simulink library "eventsBswLib"  (R2023b)
settings: Solver=VariableStepAuto  StartTime=0.0  StopTime=10.0  RelTol=1e-3
libraries: simulink x3, events_bswapi x2
settings Model: Creator=Professional  LastModifiedBy=zon07
settings SFSimCC: SimAnalyzeCustomCode=on  SimTargetLang=C++
settings RTWCC: RTWUseSimCustomCode=on

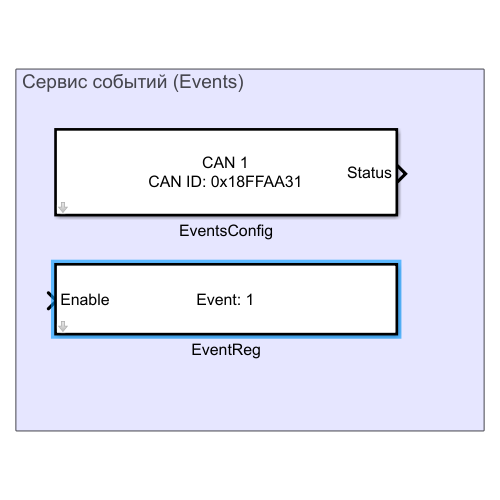
[thumbnail: Simulink's stored preview of the top-level diagram]
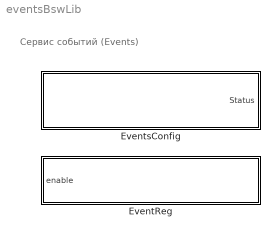
== system eventsBswLib ==
  note: Сервис событий (Events)
  EventReg : Subsystem  TreatAsAtomicUnit=on  mask(Event Registration){eventNum=1}
      mask prompts: eventNum "Номер ивента:"
      mask help:
      | Зарегистрировать ивент.
      | Активация события происходит по изменению enable из false -> true;
      | Сообщение с событием отправиться один раз.
      | Для повторной регистрации события необходимо заново перевести enable из false -> true.
      mask init:
      | blockName = "Event: " + num2str(eventNum);
      mask DialogControl Container2 Prompt: Параметры
      mask Display:
      | disp(blockName);
      | port_label('input', 1, 'Enable');
  EventsConfig : Subsystem  TreatAsAtomicUnit=on  mask(Config Events CanId){can=CAN1, canId=0x18FFAA31}
      mask prompts: canId "Events msg CanId:"
      mask help: Установить CAN ID для отправки ивентов (событий).
      mask init:
      | blockName = "CAN " + can + "\n" + "CAN ID: 0x" + dec2hex(canId);
      mask TypeOptions can: CAN1 | CAN2
      mask DialogControl ParameterGroupVar Prompt: Параметры
      mask Display:
      | disp(blockName);
      | port_label('output', 1, 'Status');

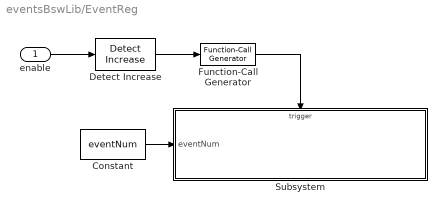
== system eventsBswLib/EventReg ==
  enable : Inport  OutDataTypeStr=boolean
  Constant : Constant  Value=eventNum  OutDataTypeStr=uint16
  Detect Increase : simulink/Logic and Bit Operations/Detect Increase  vinit=0.0  OutDataTypeStr=boolean
  Function-Call Generator : simulink/Ports & Subsystems/Function-Call Generator  sample_time=1  numberOfIterations=1  DisallowWideOutput=off  ShowEnablePort=on
  Subsystem : Subsystem
  wires:
  Constant/1 -> Subsystem/1(eventNum)
  enable/1 -> Detect Increase/1
  Function-Call Generator/1 -> Subsystem/Trigger
  Detect Increase/1 -> Function-Call Generator/1

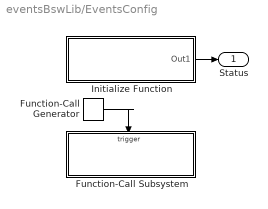
== system eventsBswLib/EventsConfig ==
  Function-Call Generator : simulink/Ports & Subsystems/Function-Call Generator  sample_time=1  numberOfIterations=1  DisallowWideOutput=off
  Function-Call Subsystem : Subsystem  TreatAsAtomicUnit=on
  Initialize Function : Subsystem  TreatAsAtomicUnit=on
  Status : Outport
  wires:
  Initialize Function/1(Out1) -> Status/1
  Function-Call Generator/1 -> Function-Call Subsystem/Trigger

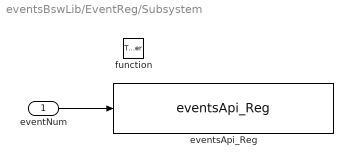
== system eventsBswLib/EventReg/Subsystem ==
  eventNum : Inport  OutDataTypeStr=uint16
  function : TriggerPort  TriggerType=function-call  VariantControl=(inherit)
  eventsApi_Reg : events_bswapi/eventsApi_Reg  SampleTime=-1
  wires:
  eventNum/1 -> eventsApi_Reg/1

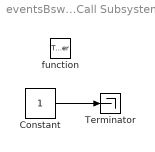
== system eventsBswLib/EventsConfig/Function-Call Subsystem ==
  function : TriggerPort  TriggerType=function-call  VariantControl=(inherit)
  Constant : Constant  OutDataTypeStr=uint8
  Terminator : Terminator
  wires:
  Constant/1 -> Terminator/1

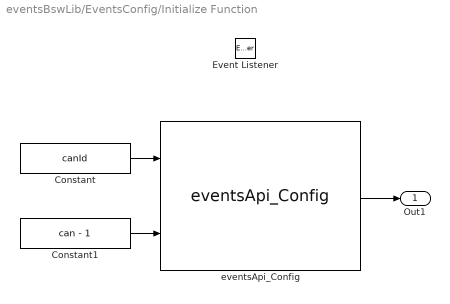
== system eventsBswLib/EventsConfig/Initialize Function ==
  Constant : Constant  Value=canId  OutDataTypeStr=uint32
  Constant1 : Constant  Value=can - 1  OutDataTypeStr=uint8
  Event Listener : EventListener  DisableCoverage=on  EventName=reset
  eventsApi_Сonfig : events_bswapi/eventsApi_Сonfig  SampleTime=-1
  Out1 : Outport
  wires:
  Constant1/1 -> eventsApi_Сonfig/2
  Constant/1 -> eventsApi_Сonfig/1
  eventsApi_Сonfig/1 -> Out1/1
